simulink model "SD2231_Lab1_2024_PIDController"  (R2023a)
settings: Solver=FixedStepAuto  StartTime=0.0  StopTime=inf  FixedStep=0.001  RelTol=1e-3  EnableMultiTasking=on
values from neighbouring files (symbols this model uses):
  K_brake = K_brake(3)    [initial_student.m]    (also in initial_student_final.m)
  K_em = K_em(3)    [initial_student.m]    (also in initial_student_final.m)
undefined symbols (not defined in the file or in its folder): DiscIntNeverNeededParam, Veh
libraries: CarMaker4SL x37, SignalEditorBlockLib x2, autolibmappedmotor x2
(part 3 of 3)

== system SD2231_Lab1_2024_PIDController/CarMaker/IPG Vehicle/CarAndTrailer/Trailer/CreateBus Vhcl.Steering ==
  In1 : Inport
  Bus Creator3 : BusCreator  Inputs=4
  Demux : Demux
      settings: DisplayOption=none
  Out1 : Outport  VectorParamsAs1DForOutWhenUnconnected=off
  wires:
  Bus Creator3/1 -> Out1/1
  Demux/1 -> Bus Creator3/1  "Vhcl Steering Ang"
  Demux/3 -> Bus Creator3/3  "Vhcl Steering AngAcc"
  Demux/2 -> Bus Creator3/2  "Vhcl Steering AngVel"
  Demux/4 -> Bus Creator3/4  "Vhcl Steering Trq"
  In1/1 -> Demux/1

== system SD2231_Lab1_2024_PIDController/CarMaker/IPG Vehicle/CarAndTrailer/Trailer/CreateBus Vhcl.Wheel.FL ==
  In1 : Inport
  Bus Creator3 : BusCreator  Inputs=14
  Demux3 : Demux  Outputs=14
      settings: DisplayOption=none
  Out1 : Outport  VectorParamsAs1DForOutWhenUnconnected=off
  wires:
  Demux3/14 -> Bus Creator3/14  "Vhcl Wheel FL Trq_WhlBearing"
  Demux3/13 -> Bus Creator3/13  "Vhcl Wheel FL Trq_T2W"
  Demux3/12 -> Bus Creator3/12  "Vhcl Wheel FL SideSlip"
  Demux3/11 -> Bus Creator3/11  "Vhcl Wheel FL LongSlip"
  Demux3/10 -> Bus Creator3/10  "Vhcl Wheel FL vBelt"
  Demux3/9 -> Bus Creator3/9  "Vhcl Wheel FL Fz"
  Demux3/8 -> Bus Creator3/8  "Vhcl Wheel FL Fy"
  Demux3/7 -> Bus Creator3/7  "Vhcl Wheel FL Fx"
  Demux3/6 -> Bus Creator3/6  "Vhcl Wheel FL r_zxy z"
  Demux3/5 -> Bus Creator3/5  "Vhcl Wheel FL r_zxy y"
  Demux3/4 -> Bus Creator3/4  "Vhcl Wheel FL r_zxy x"
  Demux3/3 -> Bus Creator3/3  "Vhcl Wheel FL t z"
  Demux3/2 -> Bus Creator3/2  "Vhcl Wheel FL t y"
  In1/1 -> Demux3/1
  Bus Creator3/1 -> Out1/1
  Demux3/1 -> Bus Creator3/1  "Vhcl Wheel FL t x"

== system SD2231_Lab1_2024_PIDController/CarMaker/IPG Vehicle/CarAndTrailer/Trailer/CreateBus Vhcl.Wheel.FR ==
  In1 : Inport
  Bus Creator3 : BusCreator  Inputs=14
  Demux3 : Demux  Outputs=14
      settings: DisplayOption=none
  Out1 : Outport  VectorParamsAs1DForOutWhenUnconnected=off
  wires:
  Demux3/14 -> Bus Creator3/14  "Vhcl Wheel FR Trq_WhlBearing"
  Demux3/13 -> Bus Creator3/13  "Vhcl Wheel FR Trq_T2W"
  Demux3/12 -> Bus Creator3/12  "Vhcl Wheel FR SideSlip"
  Demux3/11 -> Bus Creator3/11  "Vhcl Wheel FR LongSlip"
  Demux3/10 -> Bus Creator3/10  "Vhcl Wheel FR vBelt"
  Demux3/9 -> Bus Creator3/9  "Vhcl Wheel FR Fz"
  Demux3/8 -> Bus Creator3/8  "Vhcl Wheel FR Fy"
  Demux3/7 -> Bus Creator3/7  "Vhcl Wheel FR Fx"
  Demux3/6 -> Bus Creator3/6  "Vhcl Wheel FR r_zxy z"
  Demux3/5 -> Bus Creator3/5  "Vhcl Wheel FR r_zxy y"
  Demux3/4 -> Bus Creator3/4  "Vhcl Wheel FR r_zxy x"
  Demux3/3 -> Bus Creator3/3  "Vhcl Wheel FR t z"
  Demux3/2 -> Bus Creator3/2  "Vhcl Wheel FR t y"
  In1/1 -> Demux3/1
  Bus Creator3/1 -> Out1/1
  Demux3/1 -> Bus Creator3/1  "Vhcl Wheel FR t x"

== system SD2231_Lab1_2024_PIDController/CarMaker/IPG Vehicle/CarAndTrailer/Trailer/CreateBus Vhcl.Wheel.RL ==
  In1 : Inport
  Bus Creator3 : BusCreator  Inputs=14
  Demux3 : Demux  Outputs=14
      settings: DisplayOption=none
  Out1 : Outport  VectorParamsAs1DForOutWhenUnconnected=off
  wires:
  Demux3/14 -> Bus Creator3/14  "Vhcl Wheel RL Trq_WhlBearing"
  Demux3/13 -> Bus Creator3/13  "Vhcl Wheel RL Trq_T2W"
  Demux3/12 -> Bus Creator3/12  "Vhcl Wheel RL SideSlip"
  Demux3/11 -> Bus Creator3/11  "Vhcl Wheel RL LongSlip"
  Demux3/10 -> Bus Creator3/10  "Vhcl Wheel RL vBelt"
  Demux3/9 -> Bus Creator3/9  "Vhcl Wheel RL Fz"
  Demux3/8 -> Bus Creator3/8  "Vhcl Wheel RL Fy"
  Demux3/7 -> Bus Creator3/7  "Vhcl Wheel RL Fx"
  Demux3/6 -> Bus Creator3/6  "Vhcl Wheel RL r_zxy z"
  Demux3/5 -> Bus Creator3/5  "Vhcl Wheel RL r_zxy y"
  Demux3/4 -> Bus Creator3/4  "Vhcl Wheel RL r_zxy x"
  Demux3/3 -> Bus Creator3/3  "Vhcl Wheel RL t z"
  Demux3/2 -> Bus Creator3/2  "Vhcl Wheel RL t y"
  In1/1 -> Demux3/1
  Bus Creator3/1 -> Out1/1
  Demux3/1 -> Bus Creator3/1  "Vhcl Wheel RL t x"

== system SD2231_Lab1_2024_PIDController/CarMaker/IPG Vehicle/CarAndTrailer/Trailer/CreateBus Vhcl.Wheel.RR ==
  In1 : Inport
  Bus Creator3 : BusCreator  Inputs=14
  Demux3 : Demux  Outputs=14
      settings: DisplayOption=none
  Out1 : Outport  VectorParamsAs1DForOutWhenUnconnected=off
  wires:
  Demux3/14 -> Bus Creator3/14  "Vhcl Wheel RR Trq_WhlBearing"
  Demux3/13 -> Bus Creator3/13  "Vhcl Wheel RR Trq_T2W"
  Demux3/12 -> Bus Creator3/12  "Vhcl Wheel RR SideSlip"
  Demux3/11 -> Bus Creator3/11  "Vhcl Wheel RR LongSlip"
  Demux3/10 -> Bus Creator3/10  "Vhcl Wheel RR vBelt"
  Demux3/9 -> Bus Creator3/9  "Vhcl Wheel RR Fz"
  Demux3/8 -> Bus Creator3/8  "Vhcl Wheel RR Fy"
  Demux3/7 -> Bus Creator3/7  "Vhcl Wheel RR Fx"
  Demux3/6 -> Bus Creator3/6  "Vhcl Wheel RR r_zxy z"
  Demux3/5 -> Bus Creator3/5  "Vhcl Wheel RR r_zxy y"
  Demux3/4 -> Bus Creator3/4  "Vhcl Wheel RR r_zxy x"
  Demux3/3 -> Bus Creator3/3  "Vhcl Wheel RR t z"
  Demux3/2 -> Bus Creator3/2  "Vhcl Wheel RR t y"
  In1/1 -> Demux3/1
  Bus Creator3/1 -> Out1/1
  Demux3/1 -> Bus Creator3/1  "Vhcl Wheel RR t x"

== system SD2231_Lab1_2024_PIDController/CarMaker/IPG Vehicle/PowerTrain/User RearDriven PowerTrain/LR Motor ==
  Gas : Inport
  "Motor speed " : Inport  Port=2
  Mapped Motor : autolibmappedmotor/Mapped Motor  port_config=Speed  param_by=Tabulated torque-speed envelope  w_t=[ 0 500 5000 10000 16000]  T_t=[440 440 350 300 280]  torque_max=.1  power_max=30  Tc=0.02  param_loss=Single efficiency measurement  eff=100  w_eff=375  T_eff=440  Piron=0  Pbase=0  w_eff_bp=[-8000 -4000 0 4000 8000]  T_eff_bp=[0 0.03 0.06 0.09]  Temp_eff_bp=[233.15 293.15 373.15]  losses_table=[1.49 1.67 2.21 3.10; 0.42 0.69 1.14 2.03; 0.06 0.24 0.78 1.68; 0.42 0.69 1.14 2.03; 1.49 1.67 2.21 3.10]  losses_table_3d=cat(3,1.05*[1.49 1.67 2.21 3.10; 0.42 0.69 1.14 2.03; 0.06 0.24 0.78 1.68; 0.42 0.69 1.14 2.03; 1.49 1.67 2.21 3.10],[1.49 1.67 2.21 3.10; 0.42 0.69 1.14 2.03; 0.06 0.24 0.78 1.68; 0.42 0.69 1.14 2.03; 1.49 1.67 2.21 3.10],1.03*[1.49 1.67 2.21 3.10; 0.42 0.69 1.14 2.03; 0.06 0.24 0.78 1.68; 0.42 0.69 1.14 2.03; 1.49 1.67 2.21 3.10])  efficiency_table=[95 95 95 95; 95 95 95 95; 95 95 95 95; 95 95 95 95; 95 95 95 95]  efficiency_table_3d=cat(3,90*ones(5,4),95*ones(5,4),92*ones(5,4))  J=0.002  b=1e-5  omega_o=0  T_t_extended=[280 300 350 440 440 440 350 300 280]  w_t_extended=[-16000 -10000 -5000 -500 0 500 5000 10000 16000]  KLossIron=0  KLossCopper=0  x_w_eff_vec=[-8000 -4000 0 4000 8000]  x_T_eff_vec=[-0.09 -0.06 -0.03 0 0.03 0.06 0.09]  x_tmp_eff_vec=[233.15 293.15 373.15]  x_losses_mat=[3.1 2.21 1.67 1.49 1.67 2.21 3.1;2.03 1.14 0.69 0.42 0.69 1.14 2.03;1.68 0.78 0.24 0.06 0.24 0.78 1.68;2.03 1.14 0.69 0.42 0.69 1.14 2.03;3.1 2.21 1.67 1.49 1.67 2.21 3.1]  x_losses_mat_3d=cat(3,[3.255 2.3205 1.7535 1.5645 1.7535 2.3205 3.255;2.1315 1.197 0.7245 0.441 0.7245 1.197 2.1315;1.764 0.819 0.252 0.063 0.252 0.819 1.764;2.1315 1.197 0.7245 0.441 0.7245 1.197 2.1315;3.255 2.3205 1.7535 1.5645 1.7535 2.3205 3.255],[3.1 2.21 1.67 1.49 1.67 2.21 3.1;2.03 1.14 0.69 0.42 0.69 1.14 2.03;1.68 0.78 0.24 0.06 0.24 0.78 1.68;2.03 1.14 0.69 0.42 0.69 1.14 2.03;3.1 2.21 1.67 1.49 1.67 2.21 3.1],[3.193 2.2763 1.7201 1.5347 1.7201 2.2763 3.193;2.0909 1.1742 0.7107 0.4326 0.7107 1.1742 2.0909;1.7304 0.8034 0.2472 0.0618 0.2472 0.8034 1.7304;2.0909 1.1742 0.7107 0.4326 0.7107 1.1742 2.0909;3.193 2.2763 1.7201 1.5347 1.7201 2.2763 3.193])  CalLossMapData={}  CalLossWithTempMapData={}  aMode=2  RefBlkName='autolibmappedmotor/Mapped Motor'
      settings: LibrarySourceBlock=vdynlib/Powertrain/Propulsion/Mapped Motor
  "Max Torque from motor " : Constant  Value=K_em
  Product : Product  RndMeth=Zero
  Read CM Dict : CarMaker4SL/Read CM Dict  xname=PT.BattHV.Volt_oc  xsync=off  xstime=Continuous
  Scope : Scope
  Terminator : Terminator
  Terminator1 : Terminator
  Motor Trq : Outport  VectorParamsAs1DForOutWhenUnconnected=off
  wires:
  Mapped Motor/3 -> Motor Trq/1
  Read CM Dict/1 -> Mapped Motor/1
  Gas/1 -> Product/1
  Product/1 -> Mapped Motor/3
  "Max Torque from motor "/1 -> Product/2
  Mapped Motor/1 -> Terminator/1
  Mapped Motor/2 -> Terminator1/1
  "Motor speed "/1 -> Scope/1, Mapped Motor/2

== system SD2231_Lab1_2024_PIDController/CarMaker/IPG Vehicle/PowerTrain/User RearDriven PowerTrain/RR Motor ==
  Gas : Inport
  "Motor speed " : Inport  Port=2
  Mapped Motor : autolibmappedmotor/Mapped Motor  port_config=Speed  param_by=Tabulated torque-speed envelope  w_t=[ 0 500 5000 10000 16000]  T_t=[440 440 350 300 280]  torque_max=.1  power_max=30  Tc=0.02  param_loss=Single efficiency measurement  eff=100  w_eff=375  T_eff=440  Piron=0  Pbase=0  w_eff_bp=[-8000 -4000 0 4000 8000]  T_eff_bp=[0 0.03 0.06 0.09]  Temp_eff_bp=[233.15 293.15 373.15]  losses_table=[1.49 1.67 2.21 3.10; 0.42 0.69 1.14 2.03; 0.06 0.24 0.78 1.68; 0.42 0.69 1.14 2.03; 1.49 1.67 2.21 3.10]  losses_table_3d=cat(3,1.05*[1.49 1.67 2.21 3.10; 0.42 0.69 1.14 2.03; 0.06 0.24 0.78 1.68; 0.42 0.69 1.14 2.03; 1.49 1.67 2.21 3.10],[1.49 1.67 2.21 3.10; 0.42 0.69 1.14 2.03; 0.06 0.24 0.78 1.68; 0.42 0.69 1.14 2.03; 1.49 1.67 2.21 3.10],1.03*[1.49 1.67 2.21 3.10; 0.42 0.69 1.14 2.03; 0.06 0.24 0.78 1.68; 0.42 0.69 1.14 2.03; 1.49 1.67 2.21 3.10])  efficiency_table=[95 95 95 95; 95 95 95 95; 95 95 95 95; 95 95 95 95; 95 95 95 95]  efficiency_table_3d=cat(3,90*ones(5,4),95*ones(5,4),92*ones(5,4))  J=0.002  b=1e-5  omega_o=0  T_t_extended=[280 300 350 440 440 440 350 300 280]  w_t_extended=[-16000 -10000 -5000 -500 0 500 5000 10000 16000]  KLossIron=0  KLossCopper=0  x_w_eff_vec=[-8000 -4000 0 4000 8000]  x_T_eff_vec=[-0.09 -0.06 -0.03 0 0.03 0.06 0.09]  x_tmp_eff_vec=[233.15 293.15 373.15]  x_losses_mat=[3.1 2.21 1.67 1.49 1.67 2.21 3.1;2.03 1.14 0.69 0.42 0.69 1.14 2.03;1.68 0.78 0.24 0.06 0.24 0.78 1.68;2.03 1.14 0.69 0.42 0.69 1.14 2.03;3.1 2.21 1.67 1.49 1.67 2.21 3.1]  x_losses_mat_3d=cat(3,[3.255 2.3205 1.7535 1.5645 1.7535 2.3205 3.255;2.1315 1.197 0.7245 0.441 0.7245 1.197 2.1315;1.764 0.819 0.252 0.063 0.252 0.819 1.764;2.1315 1.197 0.7245 0.441 0.7245 1.197 2.1315;3.255 2.3205 1.7535 1.5645 1.7535 2.3205 3.255],[3.1 2.21 1.67 1.49 1.67 2.21 3.1;2.03 1.14 0.69 0.42 0.69 1.14 2.03;1.68 0.78 0.24 0.06 0.24 0.78 1.68;2.03 1.14 0.69 0.42 0.69 1.14 2.03;3.1 2.21 1.67 1.49 1.67 2.21 3.1],[3.193 2.2763 1.7201 1.5347 1.7201 2.2763 3.193;2.0909 1.1742 0.7107 0.4326 0.7107 1.1742 2.0909;1.7304 0.8034 0.2472 0.0618 0.2472 0.8034 1.7304;2.0909 1.1742 0.7107 0.4326 0.7107 1.1742 2.0909;3.193 2.2763 1.7201 1.5347 1.7201 2.2763 3.193])  CalLossMapData={}  CalLossWithTempMapData={}  aMode=2  RefBlkName='autolibmappedmotor/Mapped Motor'
      settings: LibrarySourceBlock=vdynlib/Powertrain/Propulsion/Mapped Motor
  "Max Torque from motor " : Constant  Value=K_em
  Product : Product  RndMeth=Zero
  Read CM Dict : CarMaker4SL/Read CM Dict  xname=PT.BattHV.Volt_oc  xsync=off  xstime=Continuous
  Scope : Scope
  Terminator : Terminator
  Terminator1 : Terminator
  Motor Trq : Outport  VectorParamsAs1DForOutWhenUnconnected=off
  wires:
  Mapped Motor/3 -> Motor Trq/1
  Read CM Dict/1 -> Mapped Motor/1
  Gas/1 -> Product/1
  Product/1 -> Mapped Motor/3
  "Max Torque from motor "/1 -> Product/2
  Mapped Motor/1 -> Terminator/1
  Mapped Motor/2 -> Terminator1/1
  "Motor speed "/1 -> Scope/1, Mapped Motor/2

== system SD2231_Lab1_2024_PIDController/CarMaker/IPG Vehicle/PowerTrain/User RearDriven PowerTrain/Subsystem ==
  LR motor Torque : Inport
  RR motor Torque : Inport  Port=2
  Gear ratio : Gain  Gain=9.73
  Gear ratio1 : Gain  Gain=9.73
  "LRTrq " : Outport  VectorParamsAs1DForOutWhenUnconnected=off
  RRTrq : Outport  Port=2  VectorParamsAs1DForOutWhenUnconnected=off
  wires:
  LR motor Torque/1 -> Gear ratio1/1
  RR motor Torque/1 -> Gear ratio/1
  Gear ratio/1 -> RRTrq/1
  Gear ratio1/1 -> "LRTrq "/1

== system SD2231_Lab1_2024_PIDController/CarMaker/IPG Vehicle/PowerTrain/User RearDriven PowerTrain/WheelInertia ==
  In1 : Inport
  Divide : Product  Inputs=*/
  Read CM Parameter : CarMaker4SL/Read CM Parameter  xfile=Vehicle  xkey=Wheel.fl.I  xnout=3  xdefaults=[]  xmuxed=off  xstime=Continuous
      settings: SourceProductName=CarMaker4SL
  Switch : Switch  Criteria=u2 ~= 0  ZeroCross=off  SaturateOnIntegerOverflow=off  InputSameDT=off
  Terminator : Terminator
  Terminator1 : Terminator
  Zero : Constant
  Out1 : Outport  VectorParamsAs1DForOutWhenUnconnected=off
  wires:
  Read CM Parameter/2 -> Switch/1, Switch/2
  Switch/1 -> Divide/2
  Zero/1 -> Switch/3
  In1/1 -> Divide/1
  Read CM Parameter/3 -> Terminator1/1
  Read CM Parameter/1 -> Terminator/1
  Divide/1 -> Out1/1

== system SD2231_Lab1_2024_PIDController/CarMaker/IPG Vehicle/PowerTrain/User RearDriven PowerTrain/WheelInertia1 ==
  In1 : Inport
  Divide : Product  Inputs=*/
  Read CM Parameter : CarMaker4SL/Read CM Parameter  xfile=Vehicle  xkey=Wheel.fr.I  xnout=3  xdefaults=[]  xmuxed=off  xstime=Continuous
      settings: SourceProductName=CarMaker4SL
  Switch : Switch  Criteria=u2 ~= 0  ZeroCross=off  SaturateOnIntegerOverflow=off  InputSameDT=off
  Terminator : Terminator
  Terminator1 : Terminator
  Zero : Constant
  Out1 : Outport  VectorParamsAs1DForOutWhenUnconnected=off
  wires:
  Divide/1 -> Out1/1
  Read CM Parameter/1 -> Terminator/1
  Read CM Parameter/3 -> Terminator1/1
  In1/1 -> Divide/1
  Read CM Parameter/2 -> Switch/2, Switch/1
  Zero/1 -> Switch/3
  Switch/1 -> Divide/2

== system SD2231_Lab1_2024_PIDController/CarMaker/IPG Vehicle/PowerTrain/User RearDriven PowerTrain/WheelInertia2 ==
  In1 : Inport
  Divide : Product  Inputs=*/
  Read CM Parameter : CarMaker4SL/Read CM Parameter  xfile=Vehicle  xkey=Wheel.rl.I  xnout=3  xdefaults=[]  xmuxed=off  xstime=Continuous
      settings: SourceProductName=CarMaker4SL
  Switch : Switch  Criteria=u2 ~= 0  ZeroCross=off  SaturateOnIntegerOverflow=off  InputSameDT=off
  Terminator : Terminator
  Terminator1 : Terminator
  Zero : Constant
  Out1 : Outport  VectorParamsAs1DForOutWhenUnconnected=off
  wires:
  Switch/1 -> Divide/2
  Zero/1 -> Switch/3
  Read CM Parameter/2 -> Switch/1, Switch/2
  In1/1 -> Divide/1
  Read CM Parameter/3 -> Terminator1/1
  Read CM Parameter/1 -> Terminator/1
  Divide/1 -> Out1/1

== system SD2231_Lab1_2024_PIDController/CarMaker/IPG Vehicle/PowerTrain/User RearDriven PowerTrain/WheelInertia3 ==
  In1 : Inport
  Divide : Product  Inputs=*/
  Read CM Parameter : CarMaker4SL/Read CM Parameter  xfile=Vehicle  xkey=Wheel.rr.I  xnout=3  xdefaults=[]  xmuxed=off  xstime=Continuous
      settings: SourceProductName=CarMaker4SL
  Switch : Switch  Criteria=u2 ~= 0  ZeroCross=off  SaturateOnIntegerOverflow=off  InputSameDT=off
  Terminator : Terminator
  Terminator1 : Terminator
  Zero : Constant
  Out1 : Outport  VectorParamsAs1DForOutWhenUnconnected=off
  wires:
  Divide/1 -> Out1/1
  Read CM Parameter/1 -> Terminator/1
  Read CM Parameter/3 -> Terminator1/1
  In1/1 -> Divide/1
  Read CM Parameter/2 -> Switch/2, Switch/1
  Zero/1 -> Switch/3
  Switch/1 -> Divide/2

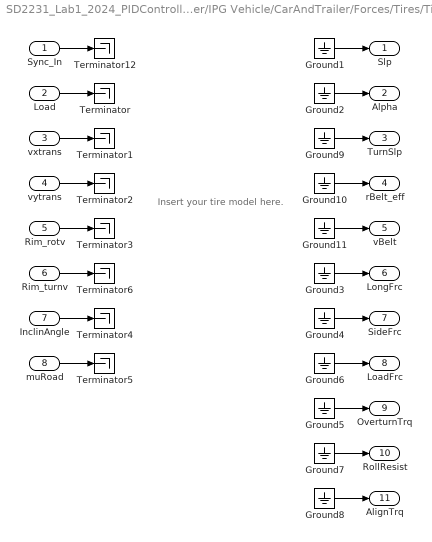
== system SD2231_Lab1_2024_PIDController/CarMaker/IPG Vehicle/CarAndTrailer/Forces/Tires/TireFL ==
  note: Insert your tire model here.
  Sync_In : Inport
  Load : Inport  Port=2
  vxtrans : Inport  Port=3
  vytrans : Inport  Port=4
  Rim_rotv : Inport  Port=5
  Rim_turnv : Inport  Port=6
  InclinAngle : Inport  Port=7
  muRoad : Inport  Port=8
  Ground{1..11} (11 alike) : Ground
  Terminator{,1..6,12} (8 alike) : Terminator
  Slp : Outport  VectorParamsAs1DForOutWhenUnconnected=off
  Alpha : Outport  Port=2  VectorParamsAs1DForOutWhenUnconnected=off
  TurnSlp : Outport  Port=3  VectorParamsAs1DForOutWhenUnconnected=off
  rBelt_eff : Outport  Port=4  VectorParamsAs1DForOutWhenUnconnected=off
  vBelt : Outport  Port=5  VectorParamsAs1DForOutWhenUnconnected=off
  LongFrc : Outport  Port=6  VectorParamsAs1DForOutWhenUnconnected=off
  SideFrc : Outport  Port=7  VectorParamsAs1DForOutWhenUnconnected=off
  LoadFrc : Outport  Port=8  VectorParamsAs1DForOutWhenUnconnected=off
  OverturnTrq : Outport  Port=9  VectorParamsAs1DForOutWhenUnconnected=off
  RollResist : Outport  Port=10  VectorParamsAs1DForOutWhenUnconnected=off
  AlignTrq : Outport  Port=11  VectorParamsAs1DForOutWhenUnconnected=off
  wires:
  Ground11/1 -> vBelt/1
  Ground10/1 -> rBelt_eff/1
  Ground9/1 -> TurnSlp/1
  Rim_turnv/1 -> Terminator6/1
  Sync_In/1 -> Terminator12/1
  Ground2/1 -> Alpha/1
  Ground3/1 -> LongFrc/1
  Ground4/1 -> SideFrc/1
  Ground5/1 -> OverturnTrq/1
  vxtrans/1 -> Terminator1/1
  vytrans/1 -> Terminator2/1
  Rim_rotv/1 -> Terminator3/1
  InclinAngle/1 -> Terminator4/1
  muRoad/1 -> Terminator5/1
  Load/1 -> Terminator/1
  Ground1/1 -> Slp/1
  Ground6/1 -> LoadFrc/1
  Ground7/1 -> RollResist/1
  Ground8/1 -> AlignTrq/1

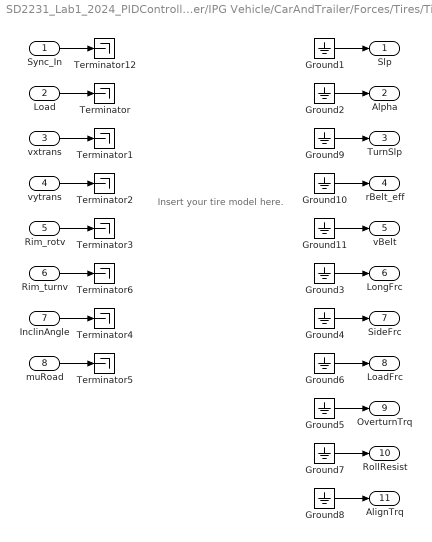
== system SD2231_Lab1_2024_PIDController/CarMaker/IPG Vehicle/CarAndTrailer/Forces/Tires/TireFR ==
  note: Insert your tire model here.
  Sync_In : Inport
  Load : Inport  Port=2
  vxtrans : Inport  Port=3
  vytrans : Inport  Port=4
  Rim_rotv : Inport  Port=5
  Rim_turnv : Inport  Port=6
  InclinAngle : Inport  Port=7
  muRoad : Inport  Port=8
  Ground{1..11} (11 alike) : Ground
  Terminator{,1..6,12} (8 alike) : Terminator
  Slp : Outport  VectorParamsAs1DForOutWhenUnconnected=off
  Alpha : Outport  Port=2  VectorParamsAs1DForOutWhenUnconnected=off
  TurnSlp : Outport  Port=3  VectorParamsAs1DForOutWhenUnconnected=off
  rBelt_eff : Outport  Port=4  VectorParamsAs1DForOutWhenUnconnected=off
  vBelt : Outport  Port=5  VectorParamsAs1DForOutWhenUnconnected=off
  LongFrc : Outport  Port=6  VectorParamsAs1DForOutWhenUnconnected=off
  SideFrc : Outport  Port=7  VectorParamsAs1DForOutWhenUnconnected=off
  LoadFrc : Outport  Port=8  VectorParamsAs1DForOutWhenUnconnected=off
  OverturnTrq : Outport  Port=9  VectorParamsAs1DForOutWhenUnconnected=off
  RollResist : Outport  Port=10  VectorParamsAs1DForOutWhenUnconnected=off
  AlignTrq : Outport  Port=11  VectorParamsAs1DForOutWhenUnconnected=off
  wires:
  Ground11/1 -> vBelt/1
  Ground10/1 -> rBelt_eff/1
  Ground9/1 -> TurnSlp/1
  Rim_turnv/1 -> Terminator6/1
  Sync_In/1 -> Terminator12/1
  Ground2/1 -> Alpha/1
  Ground3/1 -> LongFrc/1
  Ground4/1 -> SideFrc/1
  Ground5/1 -> OverturnTrq/1
  vxtrans/1 -> Terminator1/1
  vytrans/1 -> Terminator2/1
  Rim_rotv/1 -> Terminator3/1
  InclinAngle/1 -> Terminator4/1
  muRoad/1 -> Terminator5/1
  Load/1 -> Terminator/1
  Ground1/1 -> Slp/1
  Ground6/1 -> LoadFrc/1
  Ground7/1 -> RollResist/1
  Ground8/1 -> AlignTrq/1

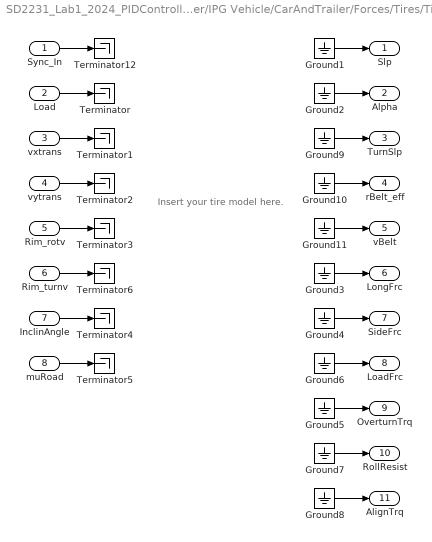
== system SD2231_Lab1_2024_PIDController/CarMaker/IPG Vehicle/CarAndTrailer/Forces/Tires/TireRL ==
  note: Insert your tire model here.
  Sync_In : Inport
  Load : Inport  Port=2
  vxtrans : Inport  Port=3
  vytrans : Inport  Port=4
  Rim_rotv : Inport  Port=5
  Rim_turnv : Inport  Port=6
  InclinAngle : Inport  Port=7
  muRoad : Inport  Port=8
  Ground{1..11} (11 alike) : Ground
  Terminator{,1..6,12} (8 alike) : Terminator
  Slp : Outport  VectorParamsAs1DForOutWhenUnconnected=off
  Alpha : Outport  Port=2  VectorParamsAs1DForOutWhenUnconnected=off
  TurnSlp : Outport  Port=3  VectorParamsAs1DForOutWhenUnconnected=off
  rBelt_eff : Outport  Port=4  VectorParamsAs1DForOutWhenUnconnected=off
  vBelt : Outport  Port=5  VectorParamsAs1DForOutWhenUnconnected=off
  LongFrc : Outport  Port=6  VectorParamsAs1DForOutWhenUnconnected=off
  SideFrc : Outport  Port=7  VectorParamsAs1DForOutWhenUnconnected=off
  LoadFrc : Outport  Port=8  VectorParamsAs1DForOutWhenUnconnected=off
  OverturnTrq : Outport  Port=9  VectorParamsAs1DForOutWhenUnconnected=off
  RollResist : Outport  Port=10  VectorParamsAs1DForOutWhenUnconnected=off
  AlignTrq : Outport  Port=11  VectorParamsAs1DForOutWhenUnconnected=off
  wires:
  Ground11/1 -> vBelt/1
  Ground10/1 -> rBelt_eff/1
  Ground9/1 -> TurnSlp/1
  Rim_turnv/1 -> Terminator6/1
  Sync_In/1 -> Terminator12/1
  Ground2/1 -> Alpha/1
  Ground3/1 -> LongFrc/1
  Ground4/1 -> SideFrc/1
  Ground5/1 -> OverturnTrq/1
  vxtrans/1 -> Terminator1/1
  vytrans/1 -> Terminator2/1
  Rim_rotv/1 -> Terminator3/1
  InclinAngle/1 -> Terminator4/1
  muRoad/1 -> Terminator5/1
  Load/1 -> Terminator/1
  Ground1/1 -> Slp/1
  Ground6/1 -> LoadFrc/1
  Ground7/1 -> RollResist/1
  Ground8/1 -> AlignTrq/1

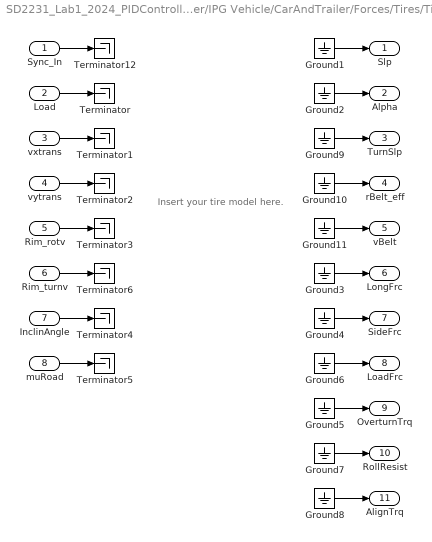
== system SD2231_Lab1_2024_PIDController/CarMaker/IPG Vehicle/CarAndTrailer/Forces/Tires/TireRR ==
  note: Insert your tire model here.
  Sync_In : Inport
  Load : Inport  Port=2
  vxtrans : Inport  Port=3
  vytrans : Inport  Port=4
  Rim_rotv : Inport  Port=5
  Rim_turnv : Inport  Port=6
  InclinAngle : Inport  Port=7
  muRoad : Inport  Port=8
  Ground{1..11} (11 alike) : Ground
  Terminator{,1..6,12} (8 alike) : Terminator
  Slp : Outport  VectorParamsAs1DForOutWhenUnconnected=off
  Alpha : Outport  Port=2  VectorParamsAs1DForOutWhenUnconnected=off
  TurnSlp : Outport  Port=3  VectorParamsAs1DForOutWhenUnconnected=off
  rBelt_eff : Outport  Port=4  VectorParamsAs1DForOutWhenUnconnected=off
  vBelt : Outport  Port=5  VectorParamsAs1DForOutWhenUnconnected=off
  LongFrc : Outport  Port=6  VectorParamsAs1DForOutWhenUnconnected=off
  SideFrc : Outport  Port=7  VectorParamsAs1DForOutWhenUnconnected=off
  LoadFrc : Outport  Port=8  VectorParamsAs1DForOutWhenUnconnected=off
  OverturnTrq : Outport  Port=9  VectorParamsAs1DForOutWhenUnconnected=off
  RollResist : Outport  Port=10  VectorParamsAs1DForOutWhenUnconnected=off
  AlignTrq : Outport  Port=11  VectorParamsAs1DForOutWhenUnconnected=off
  wires:
  Ground11/1 -> vBelt/1
  Ground10/1 -> rBelt_eff/1
  Ground9/1 -> TurnSlp/1
  Rim_turnv/1 -> Terminator6/1
  Sync_In/1 -> Terminator12/1
  Ground2/1 -> Alpha/1
  Ground3/1 -> LongFrc/1
  Ground4/1 -> SideFrc/1
  Ground5/1 -> OverturnTrq/1
  vxtrans/1 -> Terminator1/1
  vytrans/1 -> Terminator2/1
  Rim_rotv/1 -> Terminator3/1
  InclinAngle/1 -> Terminator4/1
  muRoad/1 -> Terminator5/1
  Load/1 -> Terminator/1
  Ground1/1 -> Slp/1
  Ground6/1 -> LoadFrc/1
  Ground7/1 -> RollResist/1
  Ground8/1 -> AlignTrq/1
